simulink model "test3_1"  (R2018b)
settings: Solver=VariableStepAuto  StartTime=0.0  StopTime=Endtime  RelTol=1e-3
values from neighbouring files (symbols this model uses):
  C = D ^2 / 4 *pi    (= 0.196349540849)    [TankModel.m]
  q1 = 1e-3    (= 0.001)    [TankModel.m]
  R = 500    [TankModel.m]
  smp = 0.01    [TankModel.m]
settings Model: Creator=nharada  LastModifiedBy=nharada

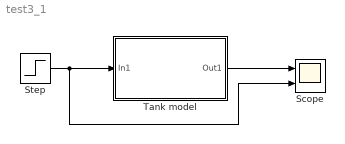
== system test3_1 ==
  Scope : Scope  NumInputPorts=2
  Step : Step  After=q1  SampleTime=smp
  "Tank model " : Subsystem
  wires:
  Step/1 -> Scope/2, "Tank model "/1(In1)
  "Tank model "/1(Out1) -> Scope/1

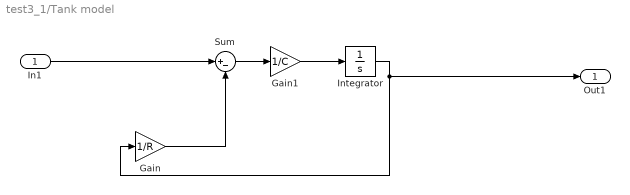
== system test3_1/Tank model  ==
  In1 : Inport
  Gain : Gain  Gain=1/R
  Gain1 : Gain  Gain=1/C
  Integrator : Integrator
  Sum : Sum  Inputs=|+-
  Out1 : Outport
  wires:
  In1/1 -> Sum/1
  Gain1/1 -> Integrator/1
  Integrator/1 -> Out1/1, Gain/1
  Sum/1 -> Gain1/1
  Gain/1 -> Sum/2
